simulink model "MMC_Single"  (R2023b)
settings: Solver=ode23tb  StartTime=0.0  StopTime=10  FixedStep=Ts_Power  RelTol=1e-3  AbsTol=1e-2
PreLoadFcn:
  | my_MMC_param
values from neighbouring files (symbols this model uses):
  Cdc_perKm = 1.4e-8    (= 1.4e-08)    [my_MMC_param.m]
  Fnom = 50    [my_MMC_param.m]
  GFL_DVC = 2    [Analysis_Main.m]    (also in initSimu.m; my_MMC_param.m)
  GFM_VF = 0    [my_MMC_param.m]
  L_cable = 15e-3 * 20    (= 0.3)    [my_MMC_param.m]
  Ldc_perKm = 2e-4    (= 0.0002)    [my_MMC_param.m]
  Ldc_r = 60e-3    (= 0.06)    [my_MMC_param.m]
  Lxfo = 0.16    [my_MMC_param.m]
  MMC1 = MMC    [Analysis_Main.m]    (also in initSimu.m)
  Pnom = 1000e6    (= 1000000000)    [my_MMC_param.m]
  R_cable = 0.5 * 5    (= 2.5)    [my_MMC_param.m]
  R_startup = 400    [my_MMC_param.m]
  Rdc_perKm = 3.3e-3    (= 0.0033)    [my_MMC_param.m]
  Rxfo = 0.002    [my_MMC_param.m]
  SEQUENCE_NO = 1    [Analysis_Main.m]    (also in initSimu.m; my_MMC_Modeling.m = 0,)
  Ton_Converter2 = 4    [my_MMC_param.m]
  Ton_PQreg = 4    [my_MMC_param.m]
  Ts_Control = Ts_Power*2    (= 0.0002)    [my_MMC_param.m]
  Ts_Power = 20e-6 * 5    (= 0.0001)    [my_MMC_param.m]
  Vnom_dc = 640e3    (= 640000)    [my_MMC_param.m]
  Vnom_prim = 400e3    (= 400000)    [my_MMC_param.m]
  Vnom_sec = 320e3    (= 320000)    [my_MMC_param.m]
  X_R = 10    [my_MMC_param.m]
undefined symbols (not defined in the file or in its folder): gcbh, Pcc, sps, sps_rtmsupport
libraries: spsSeriesRLCBranchLib x12, spsThreePhaseBreakerLib x8, spsThreePhaseSeriesRLCBranchLib x8, spsIdealSwitchLib x6, spsThreePhaseSourceLib x5, spsControlledVoltageSourceLib x4, spsPiSectionLineLib x4, spsFourierLib x3, spsGroundLib x3, simulink x2, spsPowerPositiveSequenceLib x2, spsThreePhaseTransformerTwoWindingsLib x2
Description:
  | The 'Model  initialization function' defined in the
  | 
  | Model Properties automatically sets the sample time
  | 
  | Ts to 50e-6 s
  | 
  | 
  | Copyright 2008-2016 The MathWorks, Inc.
settings Model: FPTRunName=Active  SimulationMode=accelerator  Creator=MathWorks  LastModifiedBy=uk081705
settings SolverCC: AutoScaleAbsTol=off
settings DataIOCC: SaveFormat=StructureWithTime  SaveOutput=off  DSMLogging=off  SaveTime=off  ReturnWorkspaceOutputs=off  LoggingFileName=DATA_LOG_FILE
settings OptimizationCC: BlockReduction=off  BooleanDataType=off  ExpressionDepthLimit=2147483647  InitFltsAndDblsToZero=on  EfficientMapNaN2IntZero=off  LifeSpan=inf
settings DebuggingCC: SaveWithParameterizedLinksMsg=none  UnderspecifiedInitializationDetection=Classic  MergeDetectMultiDrivingBlocksExec=none  CheckExecutionContextPreStartOutputMsg=on  SignalResolutionControl=TryResolveAllWithWarning  MultiTaskDSMMsg=warning  MultiTaskCondExecSysMsg=none  FcnCallInpInsideContextMsg=warning  StateNameClashWarn=warning  SFUnexpectedBacktrackingDiag=warning  SFNoUnconditionalDefaultTransitionDiag=warning  SFExecutionAtInitializationDiag=none  ArithmeticOperatorsInVariantConditions=warning
settings HardwareCC: ProdBitPerPointer=32  ProdBitPerSizeT=32  ProdBitPerPtrDiffT=32  ProdLargestAtomicFloat=None  ProdIntDivRoundTo=Undefined  ProdEndianess=Unspecified  ProdWordSize=32  ProdHWDeviceType=32-bit Generic  TargetBitPerPointer=64  TargetBitPerSizeT=64  TargetBitPerPtrDiffT=64  TargetLongLongMode=on  TargetIntDivRoundTo=Zero  TargetEndianess=LittleEndian  TargetWordSize=64  TargetHWDeviceType=MATLAB Host  ProdEqTarget=off
settings ModelReferenceCC: EnableRefExpFcnMdlSchedulingChecks=on  PropagateSignalLabelsOutOfModel=off
settings SFSimCC: SimUseLocalCustomCode=off  CustomCodeUndefinedFunction=UseInterfaceOnly
settings CodeAppCC: MaxIdLength=128
settings GRTTargetCC: CombineOutputUpdateFcns=off  GRTInterface=on
settings ConfigComp: CovMetricSettings=dw  CovSaveCumulativeToWorkspaceVar=on  CovSaveSingleToWorkspaceVar=on  CovExternalEMLEnable=off  CovSFcnEnable=off
settings SimscapeCC: SimscapeNormalizeSystem=off

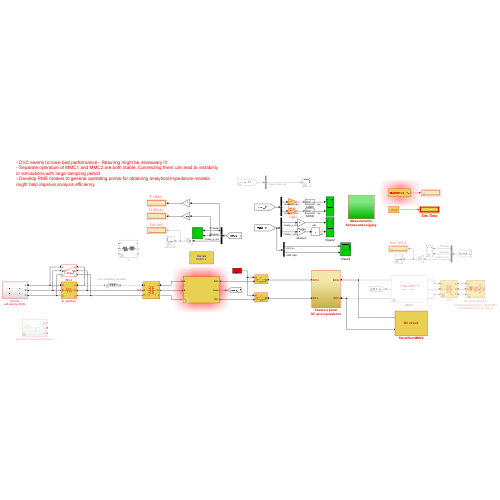
[thumbnail: Simulink's stored preview of the top-level diagram]
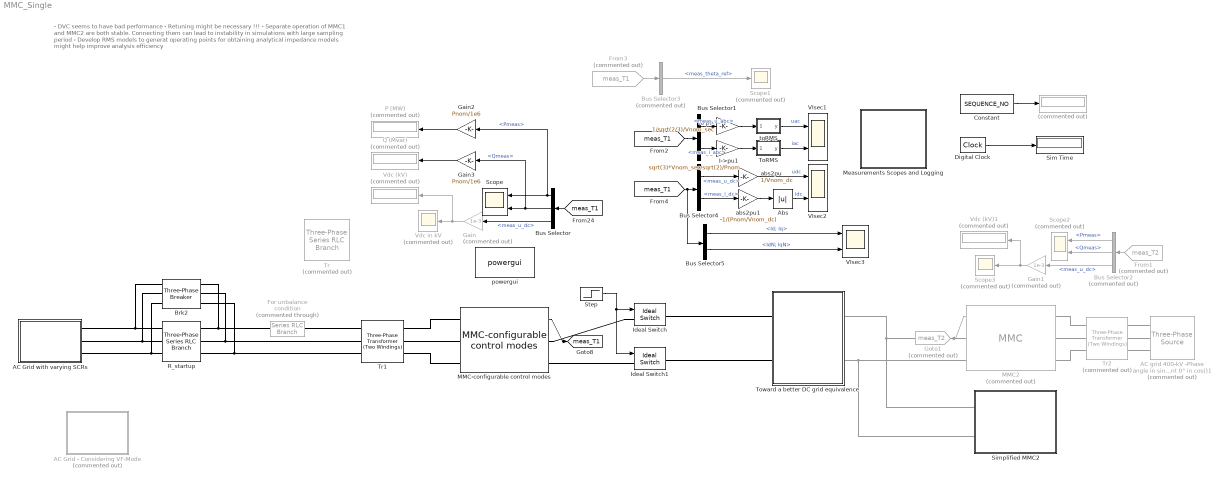
== system MMC_Single ==
  note: - DVC seems to have bad performance - Retuning might be necessary !!!
      | - Separate operation of MMC1 and MMC2 are both stable. Connecting them can lead to instability in simulations with large sampling period
      | - Develop RMS models to generat operating points for obtaining analytical impedance models might help improve analysis efficiency
  "   " : Display  Commented=on
      settings: Format=bank  Decimation=500
  AC Grid with varying SCRs : Subsystem
  AC Grid - Considering VF-Mode : Subsystem  Commented=on
  AC grid 400-kV -Phase angle in sin() with 90° to represent 0° in cos()1 : spsThreePhaseSourceLib/Three-Phase Source  Commented=on  InternalConnection=Yg  VoltagePhases=off  Voltage=Vnom_prim*1.0  PhaseAngle=90  Voltage_phases=[25e3 25e3 25e3]/sqrt(3)  PhaseAngles_phases=[0 -120 +120]  Frequency=Fnom  NonIdealSource=on  SpecifyImpedance=on  Resistance=0.8929  Inductance=16.58e-3  ShortCircuitLevel=Psc  BaseVoltage=Vnom_prim  XRratio=X_R  BusType=swing  Pref=0  Qref=0  Prefabc=[10e3, 10e3, 10e3]  Qrefabc=[0, 0, 0]  Qmin=-inf  Qmax=inf
  Abs : Abs  SaturateOnIntegerOverflow=off
  Brk2 : spsThreePhaseBreakerLib/Three-Phase Breaker  InitialState=open  SwitchA=on  SwitchB=on  SwitchC=on  SwitchTimes=Tdeblock  External=off  BreakerResistance=1e-6  SnubberResistance=1e6  SnubberCapacitance=inf  Measurements=None
  Bus Selector : BusSelector  OutputSignals=meas_out.Pmeas,meas_out.Qmeas,meas_in.meas_u_dc
  Bus Selector1 : BusSelector  OutputSignals=meas_in.meas_u_abc,meas_in.meas_i_abc
  Bus Selector2 : BusSelector  Commented=on  OutputSignals=meas_ctrl.Pmeas,meas_ctrl.Qmeas,meas_in.meas_u_dc
  Bus Selector3 : BusSelector  Commented=on  OutputSignals=meas_ctrl.meas_theta_ref
  Bus Selector4 : BusSelector  OutputSignals=meas_in.meas_u_dc,meas_in.meas_i_dc
  Bus Selector5 : BusSelector  OutputSignals=meas_out.Id; Iq,meas_out.IdN; IqN
  Constant : Constant  Value=SEQUENCE_NO
  Digital Clock : DigitalClock  SampleTime=Ts_Control
  For unbalance condition : spsSeriesRLCBranchLib/Series RLC Branch  Commented=through  LConnTagsString=__new0  RConnTagsString=__new0  BranchType=L  Resistance=1  Inductance=Vnom_prim^2 / 10e9 / (2*pi*Fnom)  SetiL0=off  InitialCurrent=0  Capacitance=1e-6  Setx0=off  InitialVoltage=0  Measurements=None
  From1 : From  Commented=on  GotoTag=meas_T2  TagVisibility=global
  From3 : From  Commented=on  GotoTag=meas_T1  TagVisibility=global
  Gain : Gain  Commented=on  Gain=1e-3
  Gain1 : Gain  Commented=on  Gain=1e-3
  Gain2 : Gain  Gain=Pnom/1e6
  Gain3 : Gain  Gain=Pnom/1e6
  Goto1 : Goto  Commented=on  GotoTag=meas_T2  TagVisibility=global
  I->pu1 : Gain  Gain=sqrt(3)*Vnom_sec/sqrt(2)/Pnom  SaturateOnIntegerOverflow=on  OutDataTypeStr=Inherit: Same as input  ParamDataTypeStr=Inherit: Same as input
  Ideal Switch : spsIdealSwitchLib/Ideal Switch  Ron=0.001  Lon=0  IC=0  Rs=1e6  Cs=inf  Measurements=off
  Ideal Switch1 : spsIdealSwitchLib/Ideal Switch  Ron=0.001  Lon=0  IC=0  Rs=1e6  Cs=inf  Measurements=off
  MMC-configurable control modes : lib_dGrid/MMC-configurable control modes  CtrlMode=MMC1.CtrlMode  Ctrl=MMC1.Ctrl  Set=MMC1.Set
      link override MMC Control/Current Regulator/PI regulator with anti-windup D1: Kp=Kp_Ireg/5  Ki=Ki_Ireg/5  Par_Limits=Limits_Ireg/5
      link override MMC Control/Current Regulator/PI regulator with anti-windup D2: Kp=Kp_Ireg/5  Ki=Ki_Ireg/5  Par_Limits=Limits_Ireg/5
      link override MMC Control/Current Regulator/SET 0 to Disable: Gain=1
      link override MMC Control/GFL//GFM Switching & Modulation (UCM // DM) & dq0 ->abc/NS-Flag: Gain=0
      link override "MMC Control/PLL, Measurements  and Transformation/ab0->dq0 PSNS": T1=1/(2*pi*30)
      link override MMC Control/VSM Control/VSM1/1//f1: Gain=1
      link override MMC Control/VSM Control/VSM1/Gain: Gain=Ctrl.IsPfDroopGFM
  MMC2 : Library_dynaGrid/MMC  Commented=on  CtrlMode=MMC2.CtrlMode  Ctrl=MMC2.Ctrl  Set=MMC2.Set
  Measurements Scopes and Logging : Subsystem
  "P (MW) " : Display  Commented=on
      settings: Format=bank  Decimation=5000
  Q (Mvar) : Display  Commented=on
      settings: Format=bank  Decimation=5000
  R_startup : spsThreePhaseSeriesRLCBranchLib/Three-Phase Series RLC Branch  LConnTagsString=A|B|C  RConnTagsString=A|B|C  BranchType=R  Resistance=R_startup  Inductance=Vnom_prim^2 / Pcc / (2*pi*Fnom)  Capacitance=1e-6  Measurements=None
  Scope : Scope  NumInputPorts=2
  Scope1 : Scope  Commented=on
  Scope2 : Scope  Commented=on  NumInputPorts=2
  Scope3 : Scope  Commented=on
  Sim Time : Display
      settings: Format=bank  Decimation=500
  Simplified MMC2 : Subsystem
      mask Display: disp('DC circuit')
  Step : Step  Time=Ton_Converter2  SampleTime=0
  ToRMS : Subsystem
  Toward a better DC grid equivalence : Subsystem
  Tr : spsThreePhaseSeriesRLCBranchLib/Three-Phase Series RLC Branch  Commented=on  LConnTagsString=A|B|C  RConnTagsString=A|B|C  BranchType=RL  Resistance=Rxfo*Vnom_sec^2/Pnom  Inductance=Lxfo*Vnom_sec^2/Pnom/(2*pi*Fnom)  Capacitance=1e-6  Measurements=None
  Tr1 : spsThreePhaseTransformerTwoWindingsLib/Three-Phase Transformer (Two Windings)  Winding1Connection=Yg  Winding2Connection=Y  CoreType=Three single-phase transformers  SetSaturation=off  Hysteresis=off  DataFile='hysteresis'  SetInitialFlux=off  Measurements=None  UNITS=pu  NominalPower=[ Pnom , Fnom ]  Winding1="[ Vnom_prim , Rxfo/2,  Lxfo/2 ]"  Winding2="[ Vnom_sec , Rxfo/2,  Lxfo/2 ]"  Rm=1000  Lm=1000  L0=0.5  Saturation=[ 0,0 ; 0.0024,1.2 ; 1.0,1.52 ]  InitialFluxes=[ 0.8 , -0.8 , 0.7 ]  BreakLoop=off  DiscreteSolver=Trapezoidal iterative  DataType=off  TransfoNumber=1
  Tr2 : spsThreePhaseTransformerTwoWindingsLib/Three-Phase Transformer (Two Windings)  Commented=on  Winding1Connection=Yg  Winding2Connection=Y  CoreType=Three single-phase transformers  SetSaturation=off  Hysteresis=off  DataFile='hysteresis'  SetInitialFlux=off  Measurements=None  UNITS=pu  NominalPower=[ Pnom , Fnom ]  Winding1="[ Vnom_prim , Rxfo/2,  Lxfo/2 ]"  Winding2="[ Vnom_sec , Rxfo/2,  Lxfo/2 ]"  Rm=1000  Lm=1000  L0=0.5  Saturation=[ 0,0 ; 0.0024,1.2 ; 1.0,1.52 ]  InitialFluxes=[ 0.8 , -0.8 , 0.7 ]  BreakLoop=off  DiscreteSolver=Trapezoidal iterative  DataType=off  TransfoNumber=1
  VIsec1 : Scope  NumInputPorts=2
  VIsec2 : Scope  NumInputPorts=2
  VIsec3 : Scope  NumInputPorts=2
  Vdc (kV) : Display  Commented=on
      settings: Format=bank  Decimation=5000
  Vdc (kV)1 : Display  Commented=on
      settings: Format=bank  Decimation=5000
  Vdc in kV : Scope  Commented=on
  abs2pu : Gain  Gain=1/Vnom_dc
  abs2pu1 : Gain  Gain=-1/(Pnom/Vnom_dc)
  powergui : spspowerguiLib/powergui  Priority=2  SimulationMode=Discrete  SampleTime=Ts_Power  frequency=60  Iterations=50  frequencyindice=0  Pbase=1000e6  ErrMax=1e-4  UnitsV=kV  UnitsW=MW  buscounter=0  FunctionMessages=off  echomessages=off  EnableUseOfTLC=off  CurrentSourceSwitches=off  DisableSnubberDevices=off  DisableRonSwitches=off  DisableVfSwitches=off  DisplayEquations=off  AutomaticDiscreteSolvers=off  SolverType=Tustin/Backward Euler (TBE)  Interpol=off  ExternalGateDelay=off  methode=off  Ts=0  x0status=blocks  SPID=off  SwTol=0  HookPort=off  NonlinearTolerance=1e-4  nMaxIteration=100  ContinueOnMaxIteration=off  RestoreLinks=warning  ResistiveCurrentMeasurement=off  Frange=[0:2:500]  Ylog=off  Xlog=on  ShowGrid=off  save=off  variable=ZData  structure=Iarm_A  ZoomFFT=off  StartTime=14  cycles=10  DisplayStyle=1  fundamental=50  FreqAxis=off  MaxFrequency=500  frequencyindicesteady=1  RmsSteady=1  display=off
  to pu : Gain  Gain=1/sqrt(2/3)/Vnom_sec
  toRMS : Subsystem
  tag scope: meas_T1=global
  wires:
  [meas_T1] -> Bus Selector/1
  MMC-configurable control modes/1 -> [meas_T1]
  Bus Selector/3 -> Gain/1  "<meas_u_dc>"
  Bus Selector/2 -> Gain3/1, Scope/2  "<Qmeas>"
  Bus Selector/1 -> Gain2/1, Scope/1  "<Pmeas>"
  Step/1 -> Ideal Switch/1, Ideal Switch1/1
  Gain/1 -> Vdc in kV/1, Vdc (kV)/1
  MMC2/1 -> Goto1/1
  Bus Selector2/3 -> Gain1/1  "<meas_u_dc>"
  From1/1 -> Bus Selector2/1
  Gain1/1 -> Scope3/1, Vdc (kV)1/1
  Bus Selector2/1 -> Scope2/1  "<Pmeas>"
  Bus Selector2/2 -> Scope2/2  "<Qmeas>"
  Digital Clock/1 -> Sim Time/1
  Constant/1 -> "   "/1
  ToRMS/1(y) -> VIsec1/2  "iac"
  to pu/1 -> toRMS/1(PhN)
  toRMS/1(y) -> VIsec1/1  "uac"
  I->pu1/1 -> ToRMS/1(PhN)
  Bus Selector1/1 -> to pu/1  "<meas_u_abc>"
  Bus Selector1/2 -> I->pu1/1  "<meas_i_abc>"
  [meas_T1] -> Bus Selector1/1
  From3/1 -> Bus Selector3/1
  Bus Selector3/1 -> Scope1/1  "<meas_theta_ref>"
  [meas_T1] -> Bus Selector5/1, Bus Selector4/1
  Bus Selector4/1 -> abs2pu/1  "<meas_u_dc>"
  abs2pu/1 -> VIsec2/1  "udc"
  Bus Selector4/2 -> abs2pu1/1  "<meas_i_dc>"
  abs2pu1/1 -> Abs/1
  Gain2/1 -> "P (MW) "/1
  Gain3/1 -> Q (Mvar)/1
  Abs/1 -> VIsec2/2  "idc"
  Bus Selector5/2 -> VIsec3/2  "<IdN; IqN>"
  Bus Selector5/1 -> VIsec3/1  "<Id; Iq>"
  connections:
  MMC2/RConn2 -- Simplified MMC2/LConn2 -- Toward a better DC grid equivalence/RConn2
  Tr2/RConn2 -- MMC2/LConn2
  Tr2/RConn1 -- MMC2/LConn1
  Tr2/RConn3 -- MMC2/LConn3
  AC grid 400-kV -Phase angle in sin() with 90° to represent 0° in cos()1/RConn1 -- Tr2/LConn1
  AC grid 400-kV -Phase angle in sin() with 90° to represent 0° in cos()1/RConn2 -- Tr2/LConn2
  AC grid 400-kV -Phase angle in sin() with 90° to represent 0° in cos()1/RConn3 -- Tr2/LConn3
  MMC-configurable control modes/LConn1 -- Tr1/RConn1
  MMC-configurable control modes/LConn2 -- Tr1/RConn2
  MMC-configurable control modes/LConn3 -- Tr1/RConn3
  R_startup/LConn1 -- AC Grid with varying SCRs/RConn1 -- Brk2/LConn1
  Brk2/RConn1 -- R_startup/RConn1 -- For unbalance condition/LConn1
  R_startup/LConn3 -- AC Grid with varying SCRs/RConn3 -- Brk2/LConn3
  R_startup/LConn2 -- AC Grid with varying SCRs/RConn2 -- Brk2/LConn2
  Brk2/RConn2 -- Tr1/LConn2 -- R_startup/RConn2
  R_startup/RConn3 -- Tr1/LConn3 -- Brk2/RConn3
  Toward a better DC grid equivalence/LConn2 -- Ideal Switch1/RConn1
  Ideal Switch/RConn1 -- Toward a better DC grid equivalence/LConn1
  MMC2/RConn1 -- Toward a better DC grid equivalence/RConn1 -- Simplified MMC2/LConn1
  Ideal Switch1/LConn1 -- MMC-configurable control modes/RConn2
  Ideal Switch/LConn1 -- MMC-configurable control modes/RConn1
  For unbalance condition/RConn1 -- Tr1/LConn1

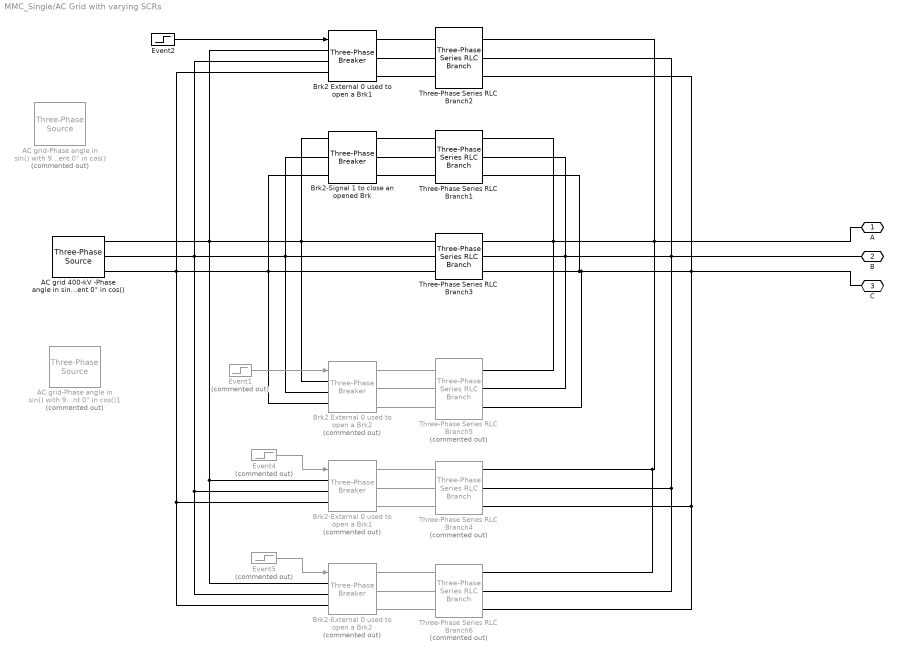
== system MMC_Single/AC Grid with varying SCRs ==
  AC grid 400-kV -Phase angle in sin() with 90° to represent 0° in cos() : spsThreePhaseSourceLib/Three-Phase Source  InternalConnection=Yg  VoltagePhases=off  Voltage=Vnom_prim*1.0  PhaseAngle=90  Voltage_phases=[25e3 25e3 25e3]/sqrt(3)  PhaseAngles_phases=[0 -120 +120]  Frequency=Fnom  NonIdealSource=off  SpecifyImpedance=on  Resistance=0.8929  Inductance=16.58e-3  ShortCircuitLevel=Psc  BaseVoltage=Vnom_prim  XRratio=X_R  BusType=swing  Pref=0  Qref=0  Prefabc=[10e3, 10e3, 10e3]  Qrefabc=[0, 0, 0]  Qmin=-inf  Qmax=inf
  AC grid-Phase angle in sin() with 90° to represent 0° in cos() : spsThreePhaseSourceLib/Three-Phase Source  Commented=on  InternalConnection=Yg  VoltagePhases=off  Voltage=Vnom_prim*1.0  PhaseAngle=90  Voltage_phases=[25e3 25e3 25e3]/sqrt(3)  PhaseAngles_phases=[0 -120 +120]  Frequency=Fnom  NonIdealSource=off  SpecifyImpedance=off  Resistance=0.8929  Inductance=16.58e-3  ShortCircuitLevel=Psc  BaseVoltage=Vnom_prim  XRratio=X_R  BusType=swing  Pref=0  Qref=0  Prefabc=[10e3, 10e3, 10e3]  Qrefabc=[0, 0, 0]  Qmin=-inf  Qmax=inf
  AC grid-Phase angle in sin() with 90° to represent 0° in cos()1 : spsThreePhaseSourceLib/Three-Phase Source  Commented=on  InternalConnection=Yg  VoltagePhases=off  Voltage=Vnom_prim*1.0  PhaseAngle=90  Voltage_phases=[25e3 25e3 25e3]/sqrt(3)  PhaseAngles_phases=[0 -120 +120]  Frequency=Fnom  NonIdealSource=on  SpecifyImpedance=on  Resistance=0.8929  Inductance=16.58e-3  ShortCircuitLevel=Psc  BaseVoltage=Vnom_prim  XRratio=X_R  BusType=swing  Pref=0  Qref=0  Prefabc=[10e3, 10e3, 10e3]  Qrefabc=[0, 0, 0]  Qmin=-inf  Qmax=inf
  Brk2 External 0 used to open a Brk1 : spsThreePhaseBreakerLib/Three-Phase Breaker  InitialState=open  SwitchA=on  SwitchB=on  SwitchC=on  SwitchTimes=7  External=on  BreakerResistance=1e-6  SnubberResistance=1e6  SnubberCapacitance=inf  Measurements=None
  Brk2 External 0 used to open a Brk2 : spsThreePhaseBreakerLib/Three-Phase Breaker  Commented=on  InitialState=closed  SwitchA=on  SwitchB=on  SwitchC=on  SwitchTimes=7  External=on  BreakerResistance=1e-6  SnubberResistance=1e6  SnubberCapacitance=inf  Measurements=None
  Brk2-External 0 used to open a Brk1 : spsThreePhaseBreakerLib/Three-Phase Breaker  Commented=on  InitialState=closed  SwitchA=on  SwitchB=on  SwitchC=on  SwitchTimes=8  External=on  BreakerResistance=1e-6  SnubberResistance=1e6  SnubberCapacitance=inf  Measurements=None
  Brk2-External 0 used to open a Brk2 : spsThreePhaseBreakerLib/Three-Phase Breaker  Commented=on  InitialState=closed  SwitchA=on  SwitchB=on  SwitchC=on  SwitchTimes=8  External=on  BreakerResistance=1e-6  SnubberResistance=1e6  SnubberCapacitance=inf  Measurements=None
  Brk2-Signal 1 to close an opened Brk : spsThreePhaseBreakerLib/Three-Phase Breaker  InitialState=open  SwitchA=on  SwitchB=on  SwitchC=on  SwitchTimes=[0 3]  External=off  BreakerResistance=1e-6  SnubberResistance=1e6  SnubberCapacitance=inf  Measurements=None
  Event1 : Step  Commented=on  Time=9  Before=1  After=0  SampleTime=0
  Event2 : Step  Time=6  SampleTime=0
  Event4 : Step  Commented=on  Time=8  Before=1  After=0  SampleTime=0
  Event5 : Step  Commented=on  Time=7  Before=1  After=0  SampleTime=0
  Three-Phase Series RLC Branch1 : spsThreePhaseSeriesRLCBranchLib/Three-Phase Series RLC Branch  LConnTagsString=A|B|C  RConnTagsString=A|B|C  BranchType=RL  Resistance=Vnom_prim^2 / 5e9 / X_R  Inductance=Vnom_prim^2 / 5e9 / (2*pi*Fnom)  Capacitance=0  Measurements=None
  Three-Phase Series RLC Branch2 : spsThreePhaseSeriesRLCBranchLib/Three-Phase Series RLC Branch  LConnTagsString=A|B|C  RConnTagsString=A|B|C  BranchType=RL  Resistance=Vnom_prim^2 / 2e9 / X_R  Inductance=Vnom_prim^2 / 2e9 / (2*pi*Fnom)  Capacitance=0  Measurements=None
  Three-Phase Series RLC Branch3 : spsThreePhaseSeriesRLCBranchLib/Three-Phase Series RLC Branch  LConnTagsString=A|B|C  RConnTagsString=A|B|C  BranchType=RL  Resistance=Vnom_prim^2 / 3e9 / X_R  Inductance=Vnom_prim^2 / 3e9 / (2*pi*Fnom)  Capacitance=0  Measurements=None
  Three-Phase Series RLC Branch4 : spsThreePhaseSeriesRLCBranchLib/Three-Phase Series RLC Branch  Commented=on  LConnTagsString=A|B|C  RConnTagsString=A|B|C  BranchType=RL  Resistance=Vnom_prim^2 / 0.1e9 / X_R  Inductance=Vnom_prim^2 / 0.1e9 / (2*pi*Fnom)  Capacitance=0  Measurements=None
  Three-Phase Series RLC Branch5 : spsThreePhaseSeriesRLCBranchLib/Three-Phase Series RLC Branch  Commented=on  LConnTagsString=A|B|C  RConnTagsString=A|B|C  BranchType=RL  Resistance=Vnom_prim^2 / 0.1e9 / X_R  Inductance=Vnom_prim^2 / 0.1e9 / (2*pi*Fnom)  Capacitance=0  Measurements=None
  Three-Phase Series RLC Branch6 : spsThreePhaseSeriesRLCBranchLib/Three-Phase Series RLC Branch  Commented=on  LConnTagsString=A|B|C  RConnTagsString=A|B|C  BranchType=RL  Resistance=Vnom_prim^2 / 0.2e9 / X_R  Inductance=Vnom_prim^2 / 0.2e9 / (2*pi*Fnom)  Capacitance=0  Measurements=None
  A : PMIOPort  Side=Right
  B : PMIOPort  Port=2  Side=Right
  C : PMIOPort  Port=3  Side=Right
  wires:
  Event2/1 -> Brk2 External 0 used to open a Brk1/1
  Event1/1 -> Brk2 External 0 used to open a Brk2/1
  Event4/1 -> Brk2-External 0 used to open a Brk1/1
  Event5/1 -> Brk2-External 0 used to open a Brk2/1
  connections:
  A/RConn1 -- Three-Phase Series RLC Branch6/RConn1 -- Three-Phase Series RLC Branch4/RConn1 -- Three-Phase Series RLC Branch2/RConn1 -- Three-Phase Series RLC Branch5/RConn1 -- Three-Phase Series RLC Branch3/RConn1 -- Three-Phase Series RLC Branch1/RConn1
  B/RConn1 -- Three-Phase Series RLC Branch6/RConn2 -- Three-Phase Series RLC Branch4/RConn2 -- Three-Phase Series RLC Branch2/RConn2 -- Three-Phase Series RLC Branch5/RConn2 -- Three-Phase Series RLC Branch3/RConn2 -- Three-Phase Series RLC Branch1/RConn2
  C/RConn1 -- Three-Phase Series RLC Branch6/RConn3 -- Three-Phase Series RLC Branch4/RConn3 -- Three-Phase Series RLC Branch2/RConn3 -- Three-Phase Series RLC Branch5/RConn3 -- Three-Phase Series RLC Branch3/RConn3 -- Three-Phase Series RLC Branch1/RConn3
  Brk2 External 0 used to open a Brk1/LConn1 -- Brk2-External 0 used to open a Brk2/LConn1 -- Brk2-External 0 used to open a Brk1/LConn1 -- AC grid 400-kV -Phase angle in sin() with 90° to represent 0° in cos()/RConn1 -- Brk2-Signal 1 to close an opened Brk/LConn1 -- Brk2 External 0 used to open a Brk2/LConn1 -- Three-Phase Series RLC Branch3/LConn1
  Brk2 External 0 used to open a Brk1/LConn2 -- Brk2-External 0 used to open a Brk2/LConn2 -- Brk2-External 0 used to open a Brk1/LConn2 -- AC grid 400-kV -Phase angle in sin() with 90° to represent 0° in cos()/RConn2 -- Brk2 External 0 used to open a Brk2/LConn2 -- Three-Phase Series RLC Branch3/LConn2 -- Brk2-Signal 1 to close an opened Brk/LConn2
  Brk2 External 0 used to open a Brk1/LConn3 -- Brk2-External 0 used to open a Brk2/LConn3 -- Brk2-External 0 used to open a Brk1/LConn3 -- AC grid 400-kV -Phase angle in sin() with 90° to represent 0° in cos()/RConn3 -- Brk2 External 0 used to open a Brk2/LConn3 -- Three-Phase Series RLC Branch3/LConn3 -- Brk2-Signal 1 to close an opened Brk/LConn3
  Three-Phase Series RLC Branch1/LConn1 -- Brk2-Signal 1 to close an opened Brk/RConn1
  Three-Phase Series RLC Branch1/LConn2 -- Brk2-Signal 1 to close an opened Brk/RConn2
  Three-Phase Series RLC Branch1/LConn3 -- Brk2-Signal 1 to close an opened Brk/RConn3
  Brk2 External 0 used to open a Brk1/RConn3 -- Three-Phase Series RLC Branch2/LConn3
  Brk2 External 0 used to open a Brk1/RConn2 -- Three-Phase Series RLC Branch2/LConn2
  Brk2 External 0 used to open a Brk1/RConn1 -- Three-Phase Series RLC Branch2/LConn1
  Three-Phase Series RLC Branch4/LConn1 -- Brk2-External 0 used to open a Brk1/RConn1
  Brk2 External 0 used to open a Brk2/RConn1 -- Three-Phase Series RLC Branch5/LConn1
  Three-Phase Series RLC Branch4/LConn2 -- Brk2-External 0 used to open a Brk1/RConn2
  Brk2 External 0 used to open a Brk2/RConn3 -- Three-Phase Series RLC Branch5/LConn3
  Three-Phase Series RLC Branch4/LConn3 -- Brk2-External 0 used to open a Brk1/RConn3
  Brk2 External 0 used to open a Brk2/RConn2 -- Three-Phase Series RLC Branch5/LConn2
  Three-Phase Series RLC Branch6/LConn3 -- Brk2-External 0 used to open a Brk2/RConn3
  Three-Phase Series RLC Branch6/LConn1 -- Brk2-External 0 used to open a Brk2/RConn1
  Three-Phase Series RLC Branch6/LConn2 -- Brk2-External 0 used to open a Brk2/RConn2

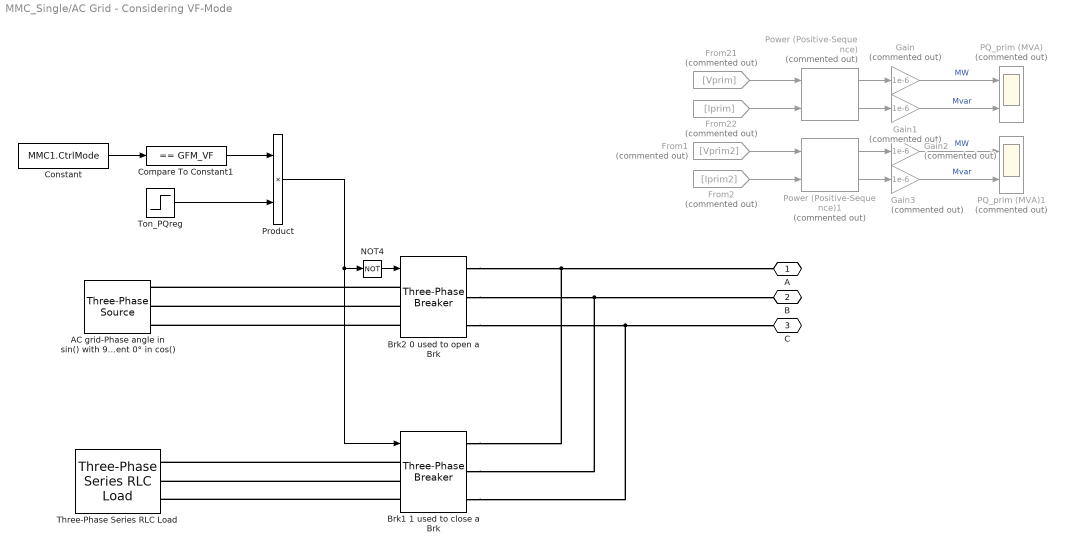
== system MMC_Single/AC Grid - Considering VF-Mode ==
  AC grid-Phase angle in sin() with 90° to represent 0° in cos() : spsThreePhaseSourceLib/Three-Phase Source  InternalConnection=Yg  VoltagePhases=off  Voltage=Vnom_prim*1.0  PhaseAngle=90  Voltage_phases=[25e3 25e3 25e3]/sqrt(3)  PhaseAngles_phases=[0 -120 +120]  Frequency=Fnom  NonIdealSource=on  SpecifyImpedance=on  Resistance=0.8929  Inductance=16.58e-3  ShortCircuitLevel=Psc  BaseVoltage=Vnom_prim  XRratio=X_R  BusType=swing  Pref=0  Qref=0  Prefabc=[10e3, 10e3, 10e3]  Qrefabc=[0, 0, 0]  Qmin=-inf  Qmax=inf
  Brk1 1 used to close a Brk : spsThreePhaseBreakerLib/Three-Phase Breaker  InitialState=open  SwitchA=on  SwitchB=on  SwitchC=on  SwitchTimes=Tdeblock  External=on  BreakerResistance=1e-6  SnubberResistance=1e6  SnubberCapacitance=inf  Measurements=None
  Brk2 0 used to open a Brk : spsThreePhaseBreakerLib/Three-Phase Breaker  InitialState=closed  SwitchA=on  SwitchB=on  SwitchC=on  SwitchTimes=Tdeblock  External=on  BreakerResistance=1e-6  SnubberResistance=1e6  SnubberCapacitance=inf  Measurements=None
  Compare To Constant1 : simulink/Logic and Bit Operations/Compare To Constant  relop===  const=GFM_VF  OutDataTypeStr=boolean
  Constant : Constant  Value=MMC1.CtrlMode
  From1 : From  Commented=on  GotoTag=Vprim2  TagVisibility=global
  From2 : From  Commented=on  GotoTag=Iprim2  TagVisibility=global
  From21 : From  Commented=on  GotoTag=Vprim  TagVisibility=global
  From22 : From  Commented=on  GotoTag=Iprim  TagVisibility=global
  Gain{,1..3} (4 alike) : Gain  Commented=on  Gain=1e-6
  NOT4 : Logic  Operator=NOT  IconShape=distinctive  AllPortsSameDT=off  OutDataTypeStr=boolean
  PQ_prim (MVA) : Scope  Commented=on  NumInputPorts=2
  PQ_prim (MVA)1 : Scope  Commented=on  NumInputPorts=2
  Power (Positive-Sequence) : spsPowerPositiveSequenceLib/Power (Positive-Sequence)  Commented=on  Freq=Fnom  Vinit=[0, 0]  Iinit=[0, 0]  Ts=Ts_Power
      settings: LibrarySourceBlock=|
      | sps_lib/Sensors and Measurements/Power
      | (Positive-Sequence)
  Power (Positive-Sequence)1 : spsPowerPositiveSequenceLib/Power (Positive-Sequence)  Commented=on  Freq=Fnom  Vinit=[0, 0]  Iinit=[0, 0]  Ts=Ts_Power
      settings: LibrarySourceBlock=|
      | sps_lib/Sensors and Measurements/Power
      | (Positive-Sequence)
  Product : Product
  Three-Phase Series RLC Load : spsThreePhaseSeriesRLCLoadLib/Three-Phase Series RLC Load  LConnTagsString=A|B|C  Configuration=Y (grounded)  NominalVoltage=Vnom_prim  Vabc=[1e3 1e3 1e3]  Vabcp=[1e3 1e3 1e3]  NominalFrequency=Fnom  UnbalancedPower=off  ActivePower=MMC1.Set.Pref*Pnom  InductivePower=100  CapacitivePower=100  Pabc=[10e3 9e3 11e3]  QLabc=[100 90 110]  QCabc=[100 90 110]  Pabcp=[10e3 9e3 11e3]  QLabcp=[100 90 110]  QCabcp=[100 90 110]  Measurements=None  LoadType=constant Z
  Ton_PQreg : Step  Time=Ton_PQreg  SampleTime=0
  A : PMIOPort  Side=Right
  B : PMIOPort  Port=2  Side=Right
  C : PMIOPort  Port=3  Side=Right
  wires:
  Compare To Constant1/1 -> Product/1
  Constant/1 -> Compare To Constant1/1
  Ton_PQreg/1 -> Product/2
  Product/1 -> Brk1 1 used to close a Brk/1, NOT4/1
  Power (Positive-Sequence)/2 -> Gain1/1
  From22/1 -> Power (Positive-Sequence)/2
  Gain/1 -> PQ_prim (MVA)/1  "MW"
  Power (Positive-Sequence)/1 -> Gain/1
  From21/1 -> Power (Positive-Sequence)/1
  Gain1/1 -> PQ_prim (MVA)/2  "Mvar"
  Gain3/1 -> PQ_prim (MVA)1/2  "Mvar"
  From1/1 -> Power (Positive-Sequence)1/1
  Power (Positive-Sequence)1/1 -> Gain2/1
  Gain2/1 -> PQ_prim (MVA)1/1  "MW"
  Power (Positive-Sequence)1/2 -> Gain3/1
  From2/1 -> Power (Positive-Sequence)1/2
  NOT4/1 -> Brk2 0 used to open a Brk/1
  connections:
  Brk2 0 used to open a Brk/RConn1 -- Brk1 1 used to close a Brk/RConn1 -- A/RConn1
  Brk2 0 used to open a Brk/RConn2 -- Brk1 1 used to close a Brk/RConn2 -- B/RConn1
  Brk2 0 used to open a Brk/RConn3 -- Brk1 1 used to close a Brk/RConn3 -- C/RConn1
  Brk2 0 used to open a Brk/LConn1 -- AC grid-Phase angle in sin() with 90° to represent 0° in cos()/RConn1
  Brk2 0 used to open a Brk/LConn2 -- AC grid-Phase angle in sin() with 90° to represent 0° in cos()/RConn2
  Brk2 0 used to open a Brk/LConn3 -- AC grid-Phase angle in sin() with 90° to represent 0° in cos()/RConn3
  Brk1 1 used to close a Brk/LConn1 -- Three-Phase Series RLC Load/LConn1
  Brk1 1 used to close a Brk/LConn2 -- Three-Phase Series RLC Load/LConn2
  Brk1 1 used to close a Brk/LConn3 -- Three-Phase Series RLC Load/LConn3

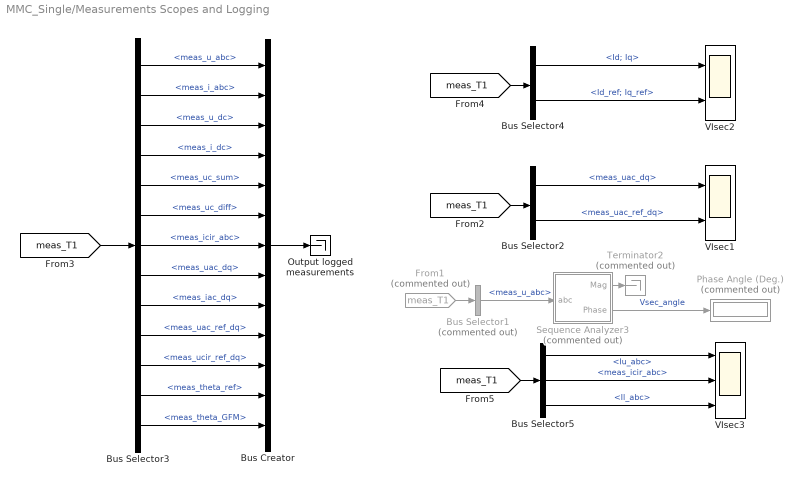
== system MMC_Single/Measurements Scopes and Logging ==
  Bus Creator : BusCreator  Inputs=13
  Bus Selector1 : BusSelector  Commented=on  OutputSignals=meas_in.meas_u_abc
  Bus Selector2 : BusSelector  OutputSignals=meas_out.meas_uac_dq,meas_out.meas_uac_ref_dq
  Bus Selector3 : BusSelector  OutputSignals=meas_in.meas_u_abc,meas_in.meas_i_abc,meas_in.meas_u_dc,meas_in.meas_i_dc,meas_out.meas_uc_sum,meas_out.meas_uc_diff,meas_out.meas_icir_abc,meas_out.meas_uac_dq,meas_out.meas_iac_dq,meas_out.meas_uac_ref_dq,meas_out.meas_ucir_ref_dq,meas_out.meas_theta_ref,meas_out.meas_theta_GFM
  Bus Selector4 : BusSelector  OutputSignals=meas_out.Id; Iq,meas_out.Id_ref; Iq_ref
  Bus Selector5 : BusSelector  OutputSignals=meas_in.Iu_abc,meas_out.meas_icir_abc,meas_in.Il_abc
  From1 : From  Commented=on  GotoTag=meas_T1  TagVisibility=global
  Output logged measurements : Terminator
  Phase Angle (Deg.) : Display  Commented=on
      settings: Format=bank
  Sequence Analyzer3 : Subsystem  Commented=on  AncestorBlock=powerlib_meascontrol/Measurements/Sequence Analyzer  DialogController=POWERSYS.PowerSysDialog  LoadFcn=sps_rtmsupport('LoadFcn', gcbh);  StartFcn=sps_rtmsupport('StartFcn', gcbh);  StopFcn=sps_rtmsupport('StopFcn', gcbh);  mask(Sequence Analyzer){Freq=Fnom, n=1, seq=Positive, InInit=[1, 0], Ts=Ts_Power}
      mask prompts: Freq "Fundamental frequency (Hz):"; n "Harmonic n (1=fundamental):"; seq "Sequence:"; InInit "Initial input [ Mag, Phase (degrees) ]:"; Ts "Sample time:"
      mask help: Compute the positive-, negative-, and zero-sequence components of a three-phase signal.
      mask init:
      | [WantBlockChoice,Ts,sps] = powericon('SequenceAnalyzerInit',gcb,Freq,n,seq,InInit,Ts);
      settings: CopyFcn=sps_rtmsupport('CopyFcn', gcbh);  DeleteFcn=sps_rtmsupport('DeleteFcn', gcbh);  UndoDeleteFcn=sps_rtmsupport('UndoDeleteFcn', gcbh);  ModelCloseFcn=sps_rtmsupport('ModelCloseFcn', gcbh);  PreSaveFcn=sps_rtmsupport('PreSaveFcn', gcbh);  PostSaveFcn=sps_rtmsupport('PostSaveFcn', gcbh);  NameChangeFcn=sps_rtmsupport('NameChangeFcn', gcbh);  PreCopyFcn=sps_rtmsupport('PreCopyFcn', gcbh);  OpenFcn=sps_rtmsupport('OpenFcn', gcbh, [3]);  CloseFcn=sps_rtmsupport('CloseFcn', gcbh);  PreDeleteFcn=sps_rtmsupport('PreDeleteFcn', gcbh);
      mask Help: helpview(psbhelp);
      mask TypeOptions seq: Positive | Negative | Zero | Positive Negative Zero
      mask Display:
      | port_label('input',1,'abc')
      | port_label('output',1,'|u|')
      | port_label('output',2,'\angleu', 'texmode', 'on')
  Terminator2 : Terminator  Commented=on
  VIsec1 : Scope  NumInputPorts=2
  VIsec2 : Scope  NumInputPorts=2
  VIsec3 : Scope  NumInputPorts=3
  wires:
  [meas_T1] -> Bus Selector3/1
  Bus Selector3/13 -> Bus Creator/13  "<meas_theta_GFM>"
  Bus Selector3/1 -> Bus Creator/1  "<meas_u_abc>"
  Bus Selector3/2 -> Bus Creator/2  "<meas_i_abc>"
  Bus Selector3/3 -> Bus Creator/3  "<meas_u_dc>"
  Bus Selector3/4 -> Bus Creator/4  "<meas_i_dc>"
  Bus Selector3/5 -> Bus Creator/5  "<meas_uc_sum>"
  Bus Selector3/6 -> Bus Creator/6  "<meas_uc_diff>"
  Bus Selector3/7 -> Bus Creator/7  "<meas_icir_abc>"
  Bus Selector3/8 -> Bus Creator/8  "<meas_uac_dq>"
  Bus Selector3/9 -> Bus Creator/9  "<meas_iac_dq>"
  Bus Selector3/10 -> Bus Creator/10  "<meas_uac_ref_dq>"
  Bus Selector3/11 -> Bus Creator/11  "<meas_ucir_ref_dq>"
  Bus Selector3/12 -> Bus Creator/12  "<meas_theta_ref>"
  Bus Creator/1 -> Output logged measurements/1
  [meas_T1] -> Bus Selector4/1
  Bus Selector4/1 -> VIsec2/1  "<Id; Iq>"
  Bus Selector4/2 -> VIsec2/2  "<Id_ref; Iq_ref>"
  Sequence Analyzer3/2(Phase) -> Phase Angle (Deg.)/1  "Vsec_angle"
  Sequence Analyzer3/1(Mag) -> Terminator2/1
  From1/1 -> Bus Selector1/1
  Bus Selector1/1 -> Sequence Analyzer3/1(abc)  "<meas_u_abc>"
  Bus Selector2/1 -> VIsec1/1  "<meas_uac_dq>"
  [meas_T1] -> Bus Selector2/1
  Bus Selector2/2 -> VIsec1/2  "<meas_uac_ref_dq>"
  [meas_T1] -> Bus Selector5/1
  Bus Selector5/2 -> VIsec3/2  "<meas_icir_abc>"
  Bus Selector5/1 -> VIsec3/1  "<Iu_abc>"
  Bus Selector5/3 -> VIsec3/3  "<Il_abc>"

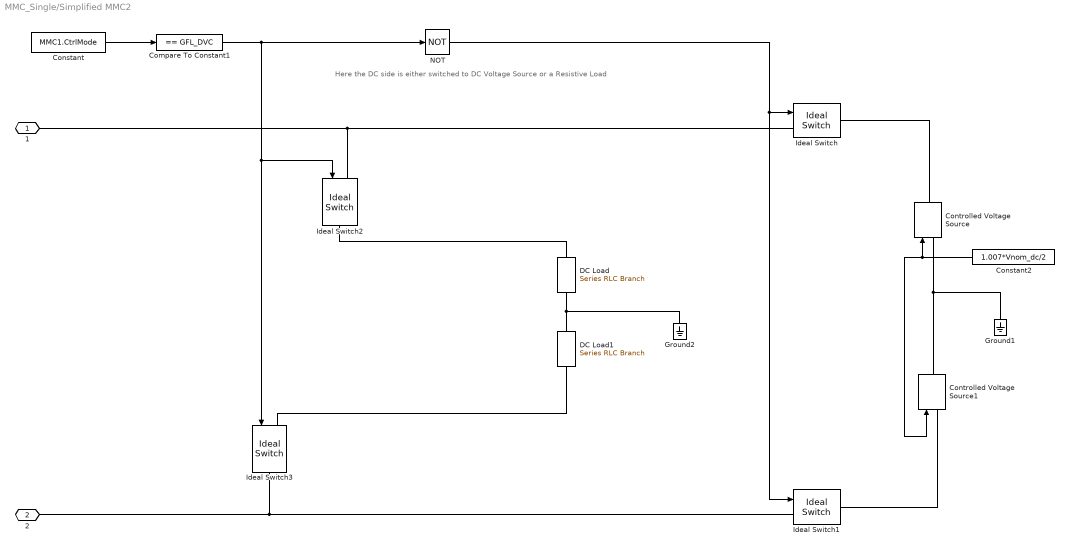
== system MMC_Single/Simplified MMC2 ==
  note: Here the DC side is either switched to DC Voltage Source or a Resistive Load
  Compare To Constant1 : simulink/Logic and Bit Operations/Compare To Constant  relop===  const=GFL_DVC  OutDataTypeStr=boolean
  Constant : Constant  Value=MMC1.CtrlMode
  Constant2 : Constant  Value=1.007*Vnom_dc/2  SampleTime=Ts_Power
  Controlled Voltage Source : spsControlledVoltageSourceLib/Controlled Voltage Source  Initialize=off  Source_Type=AC  Amplitude=0  Phase=0  Frequency=0  Measurements=None
  Controlled Voltage Source1 : spsControlledVoltageSourceLib/Controlled Voltage Source  Initialize=off  Source_Type=AC  Amplitude=0  Phase=0  Frequency=0  Measurements=None
  DC Load : spsSeriesRLCBranchLib/Series RLC Branch  LConnTagsString=__new0  RConnTagsString=__new0  BranchType=R  Resistance=(Vnom_dc/2)^2 /(MMC1.Set.Pref*Pnom/2)  Inductance=L_cable*1e2  SetiL0=off  InitialCurrent=0  Capacitance=1e-6  Setx0=off  InitialVoltage=0  Measurements=None
  DC Load1 : spsSeriesRLCBranchLib/Series RLC Branch  LConnTagsString=__new0  RConnTagsString=__new0  BranchType=R  Resistance=(Vnom_dc/2)^2 /(MMC1.Set.Pref*Pnom/2)  Inductance=L_cable*1e2  SetiL0=off  InitialCurrent=0  Capacitance=1e-6  Setx0=off  InitialVoltage=0  Measurements=None
  Ground1 : spsGroundLib/Ground  LConnTagsString=a
  Ground2 : spsGroundLib/Ground  LConnTagsString=a
  Ideal Switch{,1..3} (4 alike) : spsIdealSwitchLib/Ideal Switch  Ron=0.001  Lon=0  IC=0  Rs=1e6  Cs=inf  Measurements=off
  NOT : Logic  Operator=NOT  IconShape=distinctive  AllPortsSameDT=off  OutDataTypeStr=boolean
  1 : PMIOPort  Side=Left
  2 : PMIOPort  Port=2  Side=Left
  wires:
  Constant2/1 -> Controlled Voltage Source1/1, Controlled Voltage Source/1
  NOT/1 -> Ideal Switch1/1, Ideal Switch/1
  Constant/1 -> Compare To Constant1/1
  Compare To Constant1/1 -> Ideal Switch2/1, Ideal Switch3/1, NOT/1
  connections:
  Controlled Voltage Source1/RConn1 -- Ground1/LConn1 -- Controlled Voltage Source/LConn1
  Ideal Switch1/RConn1 -- Controlled Voltage Source1/LConn1
  Controlled Voltage Source/RConn1 -- Ideal Switch/RConn1
  Ideal Switch/LConn1 -- 1/RConn1 -- Ideal Switch2/LConn1
  DC Load/RConn1 -- DC Load1/LConn1 -- Ground2/LConn1
  Ideal Switch2/RConn1 -- DC Load/LConn1
  DC Load1/RConn1 -- Ideal Switch3/LConn1
  Ideal Switch1/LConn1 -- 2/RConn1 -- Ideal Switch3/RConn1

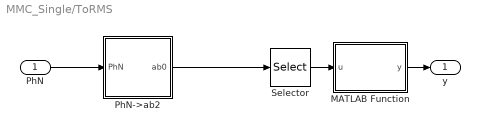
== system MMC_Single/ToRMS ==
  PhN : Inport
  MATLAB Function : MATLAB Function  TreatAsAtomicUnit=on
  PhN->ab2 : Subsystem  AncestorBlock=FriedrichLibrary/Transformations/PhN->ab0
      mask Display:
      | plot([0 1], [0,1])
      | plot([0.1 0.25 0.4 0.25 0.25], [0.5 0.6 0.5 0.6 0.8]) % Stern
      | text(0.05,1,'PhN','VerticalAlignment','Top')
      | text(0.55, 0.3,'\alpha\beta0','texmode','on')
  Selector : Selector  InputPortWidth=3  IndexOptions=Index vector (dialog)  Indices=[1 2]  OutputSizes=1
  y : Outport
  wires:
  PhN->ab2/1(ab0) -> Selector/1
  Selector/1 -> MATLAB Function/1(u)
  PhN/1 -> PhN->ab2/1(PhN)
  MATLAB Function/1(y) -> y/1

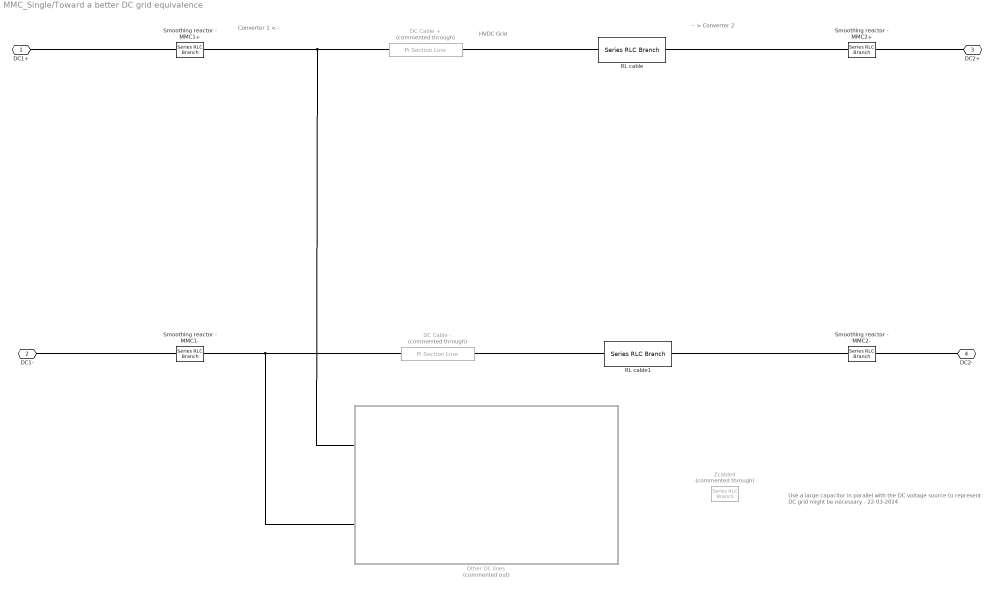
== system MMC_Single/Toward a better DC grid equivalence ==
  note: Use a large capacitor in parallel with the DC voltage source to represent DC grid might be necessary - 22-03-2024
  note: -- > Converter 2
  note: Converter 1 <--
  note: HVDC Grid
  "DC Cable + " : spsPiSectionLineLib/Pi Section Line  Commented=through  LConnTagsString=__new0  RConnTagsString=__new0  Phases=1  PiSections=1  Length=200  Frequency=Fnom  Resistance=Rdc_perKm  Inductance=Ldc_perKm  Capacitance=Cdc_perKm  SpecifyConductance=off  Conductance=0  Measurements=None  Measurements2=None
  DC Cable - : spsPiSectionLineLib/Pi Section Line  Commented=through  LConnTagsString=__new0  RConnTagsString=__new0  Phases=1  PiSections=1  Length=200  Frequency=Fnom  Resistance=Rdc_perKm  Inductance=Ldc_perKm  Capacitance=Cdc_perKm  SpecifyConductance=off  Conductance=0  Measurements=None  Measurements2=None
  Other DC lines : Subsystem  Commented=on
  RL cable : spsSeriesRLCBranchLib/Series RLC Branch  LConnTagsString=__new0  RConnTagsString=__new0  BranchType=RL  Resistance=R_cable  Inductance=L_cable  SetiL0=off  InitialCurrent=0  Capacitance=1e-6  Setx0=off  InitialVoltage=0  Measurements=None
  RL cable1 : spsSeriesRLCBranchLib/Series RLC Branch  LConnTagsString=__new0  RConnTagsString=__new0  BranchType=RL  Resistance=R_cable  Inductance=L_cable  SetiL0=off  InitialCurrent=0  Capacitance=1e-6  Setx0=off  InitialVoltage=0  Measurements=None
  Smoothing reactor - MMC1+ : spsSeriesRLCBranchLib/Series RLC Branch  LConnTagsString=__new0  RConnTagsString=__new0  BranchType=L  Resistance=1e-3  Inductance=Ldc_r  SetiL0=off  InitialCurrent=0  Capacitance=1e-6  Setx0=off  InitialVoltage=0  Measurements=None
  Smoothing reactor - MMC1- : spsSeriesRLCBranchLib/Series RLC Branch  LConnTagsString=__new0  RConnTagsString=__new0  BranchType=L  Resistance=1e-3  Inductance=Ldc_r  SetiL0=off  InitialCurrent=0  Capacitance=1e-6  Setx0=off  InitialVoltage=0  Measurements=None
  Smoothing reactor - MMC2+ : spsSeriesRLCBranchLib/Series RLC Branch  LConnTagsString=__new0  RConnTagsString=__new0  BranchType=L  Resistance=1e-3  Inductance=Ldc_r  SetiL0=off  InitialCurrent=0  Capacitance=1e-6  Setx0=off  InitialVoltage=0  Measurements=None
  Smoothing reactor - MMC2- : spsSeriesRLCBranchLib/Series RLC Branch  LConnTagsString=__new0  RConnTagsString=__new0  BranchType=L  Resistance=1e-3  Inductance=Ldc_r  SetiL0=off  InitialCurrent=0  Capacitance=1e-6  Setx0=off  InitialVoltage=0  Measurements=None
  Zcable4 : spsSeriesRLCBranchLib/Series RLC Branch  Commented=through  LConnTagsString=__new0  RConnTagsString=__new0  BranchType=R  Resistance=1e-3  Inductance=1e-3  SetiL0=off  InitialCurrent=0  Capacitance=1e-6  Setx0=off  InitialVoltage=0  Measurements=None
  DC1+ : PMIOPort  Side=Left
  DC1- : PMIOPort  Port=2  Side=Left
  DC2+ : PMIOPort  Port=3  Side=Right
  DC2- : PMIOPort  Port=4  Side=Right
  connections:
  DC1+/RConn1 -- Smoothing reactor - MMC1+/RConn1
  DC2-/RConn1 -- Smoothing reactor - MMC2-/LConn1
  DC2+/RConn1 -- Smoothing reactor - MMC2+/LConn1
  "DC Cable + "/RConn1 -- RL cable/RConn1
  RL cable1/LConn1 -- Smoothing reactor - MMC2-/RConn1
  Smoothing reactor - MMC1+/LConn1 -- "DC Cable + "/LConn1 -- Other DC lines/LConn1
  DC Cable -/LConn1 -- Other DC lines/LConn2 -- Smoothing reactor - MMC1-/LConn1
  DC1-/RConn1 -- Smoothing reactor - MMC1-/RConn1
  RL cable/LConn1 -- Smoothing reactor - MMC2+/RConn1
  RL cable1/RConn1 -- DC Cable -/RConn1

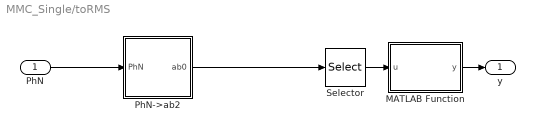
== system MMC_Single/toRMS ==
  PhN : Inport
  MATLAB Function : MATLAB Function  TreatAsAtomicUnit=on
  PhN->ab2 : Subsystem  AncestorBlock=FriedrichLibrary/Transformations/PhN->ab0
      mask Display:
      | plot([0 1], [0,1])
      | plot([0.1 0.25 0.4 0.25 0.25], [0.5 0.6 0.5 0.6 0.8]) % Stern
      | text(0.05,1,'PhN','VerticalAlignment','Top')
      | text(0.55, 0.3,'\alpha\beta0','texmode','on')
  Selector : Selector  InputPortWidth=3  IndexOptions=Index vector (dialog)  Indices=[1 2]  OutputSizes=1
  y : Outport
  wires:
  PhN->ab2/1(ab0) -> Selector/1
  Selector/1 -> MATLAB Function/1(u)
  PhN/1 -> PhN->ab2/1(PhN)
  MATLAB Function/1(y) -> y/1

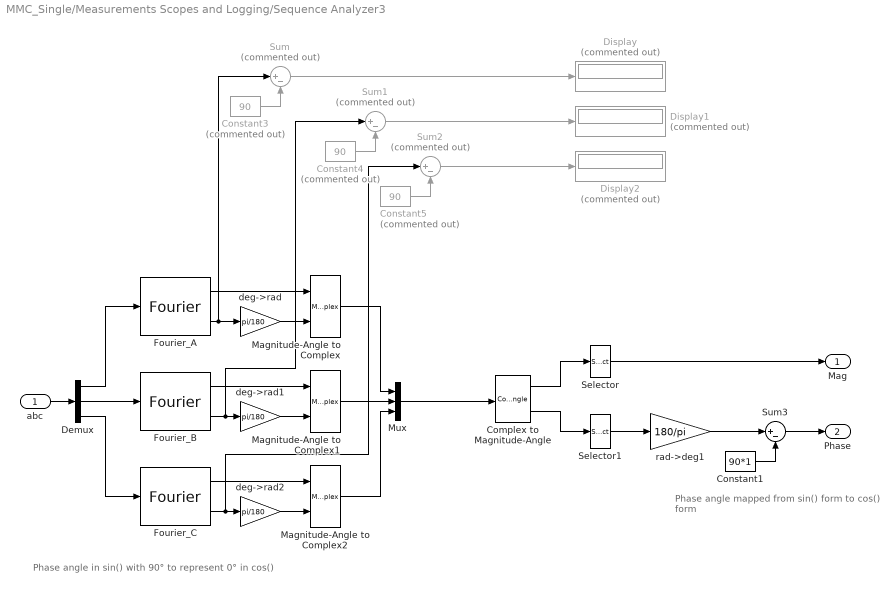
== system MMC_Single/Measurements Scopes and Logging/Sequence Analyzer3 ==
  note: Phase angle in sin() with 90° to represent 0° in cos()
  note: Phase angle mapped from sin() form to cos() form
  abc : Inport  PortDimensions=3  SampleTime=Ts
  Complex to Magnitude-Angle : ComplexToMagnitudeAngle
  Constant1 : Constant  Value=90*1
  Constant3 : Constant  Commented=on  Value=90
  Constant4 : Constant  Commented=on  Value=90
  Constant5 : Constant  Commented=on  Value=90
  Demux : Demux  Outputs=3
  Display : Display  Commented=on
  Display1 : Display  Commented=on
  Display2 : Display  Commented=on
  Fourier_A : spsFourierLib/Fourier  Freq=sps.Freq  n=sps.n  InInit=sps.Par_Init  Ts=Ts
  Fourier_B : spsFourierLib/Fourier  Freq=sps.Freq  n=sps.n  InInit="[sps.Par_Init(1)  sps.Par_Init(2)-120 ]"  Ts=Ts
  Fourier_C : spsFourierLib/Fourier  Freq=sps.Freq  n=sps.n  InInit="[sps.Par_Init(1)  sps.Par_Init(2)+120 ]"  Ts=Ts
  Magnitude-Angle to Complex : MagnitudeAngleToComplex
  Magnitude-Angle to Complex1 : MagnitudeAngleToComplex
  Magnitude-Angle to Complex2 : MagnitudeAngleToComplex
  Mux : Mux  Inputs=3
  Selector : Selector  InputPortWidth=3  IndexOptions=Index vector (dialog)  Indices=sps.SelectElement  OutputSizes=1
  Selector1 : Selector  InputPortWidth=3  IndexOptions=Index vector (dialog)  Indices=sps.SelectElement  OutputSizes=1
  Sum : Sum  Commented=on  Inputs=|+-
  Sum1 : Sum  Commented=on  Inputs=|+-
  Sum2 : Sum  Commented=on  Inputs=|+-
  Sum3 : Sum  Inputs=|+-
  deg->rad : Gain  Gain=pi/180  SaturateOnIntegerOverflow=on  OutDataTypeStr=Inherit: Same as input  ParamDataTypeStr=Inherit: Same as input
  deg->rad1 : Gain  Gain=pi/180  SaturateOnIntegerOverflow=on  OutDataTypeStr=Inherit: Same as input  ParamDataTypeStr=Inherit: Same as input
  deg->rad2 : Gain  Gain=pi/180  SaturateOnIntegerOverflow=on  OutDataTypeStr=Inherit: Same as input  ParamDataTypeStr=Inherit: Same as input
  rad->deg1 : Gain  Gain=180/pi  SaturateOnIntegerOverflow=on  OutDataTypeStr=Inherit: Same as input  ParamDataTypeStr=Inherit: Same as input
  Mag : Outport  SampleTime=Ts  InitialOutput=0  VectorParamsAs1DForOutWhenUnconnected=off
  Phase : Outport  Port=2  SampleTime=Ts  InitialOutput=0  VectorParamsAs1DForOutWhenUnconnected=off
  wires:
  Selector1/1 -> rad->deg1/1
  Magnitude-Angle to Complex2/1 -> Mux/3
  Magnitude-Angle to Complex1/1 -> Mux/2
  Magnitude-Angle to Complex/1 -> Mux/1
  Fourier_C/2 -> Sum2/1, deg->rad2/1
  deg->rad2/1 -> Magnitude-Angle to Complex2/2
  Fourier_C/1 -> Magnitude-Angle to Complex2/1
  Fourier_B/2 -> Sum1/1, deg->rad1/1
  deg->rad1/1 -> Magnitude-Angle to Complex1/2
  Fourier_B/1 -> Magnitude-Angle to Complex1/1
  deg->rad/1 -> Magnitude-Angle to Complex/2
  Fourier_A/2 -> deg->rad/1, Sum/1
  Fourier_A/1 -> Magnitude-Angle to Complex/1
  Demux/3 -> Fourier_C/1
  Demux/2 -> Fourier_B/1
  Demux/1 -> Fourier_A/1
  abc/1 -> Demux/1
  Complex to Magnitude-Angle/2 -> Selector1/1
  Selector/1 -> Mag/1
  Complex to Magnitude-Angle/1 -> Selector/1
  Mux/1 -> Complex to Magnitude-Angle/1
  Constant3/1 -> Sum/2
  Constant4/1 -> Sum1/2
  Sum1/1 -> Display1/1
  Sum/1 -> Display/1
  Constant5/1 -> Sum2/2
  Sum2/1 -> Display2/1
  Constant1/1 -> Sum3/2
  rad->deg1/1 -> Sum3/1
  Sum3/1 -> Phase/1

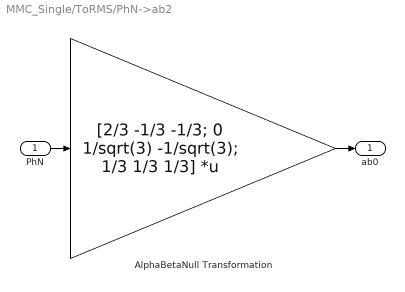
== system MMC_Single/ToRMS/PhN->ab2 ==
  PhN : Inport
  AlphaBetaNull Transformation : Gain  Gain="[2/3   -1/3    -1/3;   0   1/sqrt(3) -1/sqrt(3); 1/3 1/3 1/3]"  Multiplication=Matrix(K*u) (u vector)
  ab0 : Outport  VectorParamsAs1DForOutWhenUnconnected=off
  wires:
  AlphaBetaNull Transformation/1 -> ab0/1
  PhN/1 -> AlphaBetaNull Transformation/1

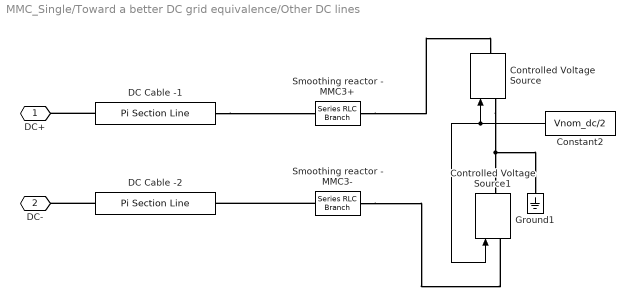
== system MMC_Single/Toward a better DC grid equivalence/Other DC lines ==
  Constant2 : Constant  Value=Vnom_dc/2  SampleTime=Ts_Power
  Controlled Voltage Source : spsControlledVoltageSourceLib/Controlled Voltage Source  Initialize=off  Source_Type=AC  Amplitude=0  Phase=0  Frequency=0  Measurements=None
  Controlled Voltage Source1 : spsControlledVoltageSourceLib/Controlled Voltage Source  Initialize=off  Source_Type=AC  Amplitude=0  Phase=0  Frequency=0  Measurements=None
  DC Cable -1 : spsPiSectionLineLib/Pi Section Line  LConnTagsString=__new0  RConnTagsString=__new0  Phases=1  PiSections=1  Length=Length_DC1  Frequency=Fnom  Resistance=Rdc_perKm  Inductance=Ldc_perKm  Capacitance=Cdc_perKm  SpecifyConductance=off  Conductance=0  Measurements=None  Measurements2=None
  DC Cable -2 : spsPiSectionLineLib/Pi Section Line  LConnTagsString=__new0  RConnTagsString=__new0  Phases=1  PiSections=1  Length=Length_DC1  Frequency=Fnom  Resistance=Rdc_perKm  Inductance=Ldc_perKm  Capacitance=Cdc_perKm  SpecifyConductance=off  Conductance=0  Measurements=None  Measurements2=None
  Ground1 : spsGroundLib/Ground  LConnTagsString=a
  Smoothing reactor - MMC3+ : spsSeriesRLCBranchLib/Series RLC Branch  LConnTagsString=__new0  RConnTagsString=__new0  BranchType=L  Resistance=1e-3  Inductance=Ldc_r  SetiL0=off  InitialCurrent=0  Capacitance=1e-6  Setx0=off  InitialVoltage=0  Measurements=None
  Smoothing reactor - MMC3- : spsSeriesRLCBranchLib/Series RLC Branch  LConnTagsString=__new0  RConnTagsString=__new0  BranchType=L  Resistance=1e-3  Inductance=Ldc_r  SetiL0=off  InitialCurrent=0  Capacitance=1e-6  Setx0=off  InitialVoltage=0  Measurements=None
  DC+ : PMIOPort  Side=Left
  DC- : PMIOPort  Port=2  Side=Left
  wires:
  Constant2/1 -> Controlled Voltage Source1/1, Controlled Voltage Source/1
  connections:
  DC Cable -2/LConn1 -- DC-/RConn1
  DC Cable -1/LConn1 -- DC+/RConn1
  DC Cable -1/RConn1 -- Smoothing reactor - MMC3+/RConn1
  Smoothing reactor - MMC3-/RConn1 -- DC Cable -2/RConn1
  Controlled Voltage Source/LConn1 -- Controlled Voltage Source1/RConn1 -- Ground1/LConn1
  Smoothing reactor - MMC3+/LConn1 -- Controlled Voltage Source/RConn1
  Smoothing reactor - MMC3-/LConn1 -- Controlled Voltage Source1/LConn1

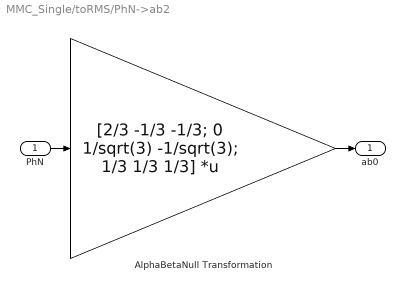
== system MMC_Single/toRMS/PhN->ab2 ==
  PhN : Inport
  AlphaBetaNull Transformation : Gain  Gain="[2/3   -1/3    -1/3;   0   1/sqrt(3) -1/sqrt(3); 1/3 1/3 1/3]"  Multiplication=Matrix(K*u) (u vector)
  ab0 : Outport  VectorParamsAs1DForOutWhenUnconnected=off
  wires:
  AlphaBetaNull Transformation/1 -> ab0/1
  PhN/1 -> AlphaBetaNull Transformation/1

== matlab function MMC_Single/toRMS/MATLAB Function ==
  data: u input; y output
function y = fcn(u)
y = sqrt(u(1)^2 + u(2)^2);

== matlab function MMC_Single/ToRMS/MATLAB Function ==
  data: u input; y output
function y = fcn(u)
y = sqrt(u(1)^2 + u(2)^2);
